simulink model "problem2"  (R2020a)
settings: Solver=VariableStepAuto  StartTime=0.0  StopTime=inf  RelTol=1e-3
settings Model: EnablePacing=on  Creator=aa  LastModifiedBy=aa

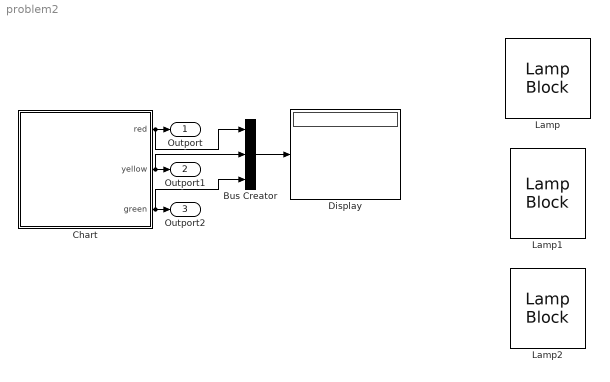
== system problem2 ==
  Bus Creator : BusCreator  Inputs=3
  Chart : Stateflow chart  TreatAsAtomicUnit=on
  Display : Display
  Lamp : LampBlock
  Lamp1 : LampBlock
  Lamp2 : LampBlock
  Outport : Outport
  Outport1 : Outport  Port=2
  Outport2 : Outport  Port=3
  wires:
  Chart/2(yellow) -> Bus Creator/2, Outport1/1
  Chart/3(green) -> Bus Creator/3, Outport2/1
  Chart/1(red) -> Bus Creator/1, Outport/1
  Bus Creator/1 -> Display/1

== stateflow chart problem2/Chart ==
  state PrepareToStop
    during:
    red=0;
    yellow=1;
    green=0;
  state Go
    during:
    red=0;
    yellow=0;
    green=1;
  state Stop
    during:
    red=1;
    yellow=0;
    green=0;
  (default) -> Stop
  Stop -> PrepareToStop : after(10,sec){state = 1;}
  PrepareToStop -> Go [order 1] : after(2,sec)[state == 1]{state=0;}
  Go -> PrepareToStop : after(30,sec)
  PrepareToStop -> Stop [order 2] : after(2,sec)
  data: red output; yellow output; green output; state local
